simulink model "RealtimeModel"  (Simulink 7.0)
settings: Solver=FixedStepDiscrete  SolverMode=MultiTasking  StartTime=0.0  StopTime=RunningTime  FixedStep=sample  RelTol=1e-3
values from neighbouring files (symbols this model uses):
  Integrator = InitializeIntegrator(Integrator, Structure)    [RealtimeModel_Setup.m]
  SampleRate = Integrator.Timestep    [RealtimeModel_Setup.m]
  Structure = CalculateMatrices(Structure, Elements)    [RealtimeModel_Setup.m]
undefined symbols (not defined in the file or in its folder): Elements
libraries: simulink x2
(part 2 of 11)

== system RealtimeModel/Generate Element  Restoring Forces/Generate Type 3  Element Restoring Force Element 2 ==
  Displ_cmd : Inport  OutDataType=sfix(16)  OutScaling=2^0
  Constant : Constant  Value=Structure.NumFreeDOF  OutDataType=sfix(16)  OutScaling=2^0
  "Type 3 Element " : Subsystem  mask(Element Type 3){id=id}
      mask prompts: id "Element ID:"
      mask help: Enter the ID for this element corresponding with the input configuration file
  Type 3 Element RF : Stateflow chart  TreatAsAtomicUnit=on  SystemSampleTime=SampleRate
  Nodes : Outport  OutDataType=sfix(16)  OutScaling=2^0
  RF : Outport  Port=2  OutDataType=sfix(16)  OutScaling=2^0
  wires:
  Constant/1 -> Type 3 Element RF/6(NumFreeDOF)
  Displ_cmd/1 -> Type 3 Element RF/7(Displacement)
  "Type 3 Element "/1(Element) -> Type 3 Element RF/1(Element)
  Type 3 Element RF/2(RF) -> RF/1
  Type 3 Element RF/1(Nodes) -> Nodes/1
  "Type 3 Element "/2(a1) -> Type 3 Element RF/2(a1)
  "Type 3 Element "/3(a2) -> Type 3 Element RF/3(a2)
  "Type 3 Element "/4(pmx) -> Type 3 Element RF/4(pmx)
  "Type 3 Element "/5(bmy) -> Type 3 Element RF/5(bmy_init)

== system RealtimeModel/Generate Element  Restoring Forces/Generate Type 3  Element Restoring Force Element 21 ==
  Displ_cmd : Inport  OutDataType=sfix(16)  OutScaling=2^0
  Constant : Constant  Value=Structure.NumFreeDOF  OutDataType=sfix(16)  OutScaling=2^0
  "Type 3 Element " : Subsystem  mask(Element Type 3){id=id}
      mask prompts: id "Element ID:"
      mask help: Enter the ID for this element corresponding with the input configuration file
  Type 3 Element RF : Stateflow chart  TreatAsAtomicUnit=on  SystemSampleTime=SampleRate
  Nodes : Outport  OutDataType=sfix(16)  OutScaling=2^0
  RF : Outport  Port=2  OutDataType=sfix(16)  OutScaling=2^0
  wires:
  "Type 3 Element "/5(bmy) -> Type 3 Element RF/5(bmy_init)
  "Type 3 Element "/4(pmx) -> Type 3 Element RF/4(pmx)
  "Type 3 Element "/3(a2) -> Type 3 Element RF/3(a2)
  "Type 3 Element "/2(a1) -> Type 3 Element RF/2(a1)
  Type 3 Element RF/1(Nodes) -> Nodes/1
  Type 3 Element RF/2(RF) -> RF/1
  "Type 3 Element "/1(Element) -> Type 3 Element RF/1(Element)
  Displ_cmd/1 -> Type 3 Element RF/7(Displacement)
  Constant/1 -> Type 3 Element RF/6(NumFreeDOF)

== system RealtimeModel/Generate Element  Restoring Forces/Generate Type 3  Element Restoring Force Element 22 ==
  Displ_cmd : Inport  OutDataType=sfix(16)  OutScaling=2^0
  Constant : Constant  Value=Structure.NumFreeDOF  OutDataType=sfix(16)  OutScaling=2^0
  "Type 3 Element " : Subsystem  mask(Element Type 3){id=id}
      mask prompts: id "Element ID:"
      mask help: Enter the ID for this element corresponding with the input configuration file
  Type 3 Element RF : Stateflow chart  TreatAsAtomicUnit=on  SystemSampleTime=SampleRate
  Nodes : Outport  OutDataType=sfix(16)  OutScaling=2^0
  RF : Outport  Port=2  OutDataType=sfix(16)  OutScaling=2^0
  wires:
  Constant/1 -> Type 3 Element RF/6(NumFreeDOF)
  Displ_cmd/1 -> Type 3 Element RF/7(Displacement)
  "Type 3 Element "/1(Element) -> Type 3 Element RF/1(Element)
  Type 3 Element RF/2(RF) -> RF/1
  Type 3 Element RF/1(Nodes) -> Nodes/1
  "Type 3 Element "/2(a1) -> Type 3 Element RF/2(a1)
  "Type 3 Element "/3(a2) -> Type 3 Element RF/3(a2)
  "Type 3 Element "/4(pmx) -> Type 3 Element RF/4(pmx)
  "Type 3 Element "/5(bmy) -> Type 3 Element RF/5(bmy_init)

== system RealtimeModel/Generate Element  Restoring Forces/Generate Type 3  Element Restoring Force Element 24 ==
  Displ_cmd : Inport  OutDataType=sfix(16)  OutScaling=2^0
  Constant : Constant  Value=Structure.NumFreeDOF  OutDataType=sfix(16)  OutScaling=2^0
  "Type 3 Element " : Subsystem  mask(Element Type 3){id=id}
      mask prompts: id "Element ID:"
      mask help: Enter the ID for this element corresponding with the input configuration file
  Type 3 Element RF : Stateflow chart  TreatAsAtomicUnit=on  SystemSampleTime=SampleRate
  Nodes : Outport  OutDataType=sfix(16)  OutScaling=2^0
  RF : Outport  Port=2  OutDataType=sfix(16)  OutScaling=2^0
  wires:
  "Type 3 Element "/5(bmy) -> Type 3 Element RF/5(bmy_init)
  "Type 3 Element "/4(pmx) -> Type 3 Element RF/4(pmx)
  "Type 3 Element "/3(a2) -> Type 3 Element RF/3(a2)
  "Type 3 Element "/2(a1) -> Type 3 Element RF/2(a1)
  Type 3 Element RF/1(Nodes) -> Nodes/1
  Type 3 Element RF/2(RF) -> RF/1
  "Type 3 Element "/1(Element) -> Type 3 Element RF/1(Element)
  Displ_cmd/1 -> Type 3 Element RF/7(Displacement)
  Constant/1 -> Type 3 Element RF/6(NumFreeDOF)

== system RealtimeModel/Generate Element  Restoring Forces/Generate Type 3  Element Restoring Force Element 25 ==
  Displ_cmd : Inport  OutDataType=sfix(16)  OutScaling=2^0
  Constant : Constant  Value=Structure.NumFreeDOF  OutDataType=sfix(16)  OutScaling=2^0
  "Type 3 Element " : Subsystem  mask(Element Type 3){id=id}
      mask prompts: id "Element ID:"
      mask help: Enter the ID for this element corresponding with the input configuration file
  Type 3 Element RF : Stateflow chart  TreatAsAtomicUnit=on  SystemSampleTime=SampleRate
  Nodes : Outport  OutDataType=sfix(16)  OutScaling=2^0
  RF : Outport  Port=2  OutDataType=sfix(16)  OutScaling=2^0
  wires:
  "Type 3 Element "/5(bmy) -> Type 3 Element RF/5(bmy_init)
  "Type 3 Element "/4(pmx) -> Type 3 Element RF/4(pmx)
  "Type 3 Element "/3(a2) -> Type 3 Element RF/3(a2)
  "Type 3 Element "/2(a1) -> Type 3 Element RF/2(a1)
  Type 3 Element RF/1(Nodes) -> Nodes/1
  Type 3 Element RF/2(RF) -> RF/1
  "Type 3 Element "/1(Element) -> Type 3 Element RF/1(Element)
  Displ_cmd/1 -> Type 3 Element RF/7(Displacement)
  Constant/1 -> Type 3 Element RF/6(NumFreeDOF)

== system RealtimeModel/Generate Element  Restoring Forces/Generate Type 3  Element Restoring Force Element 26 ==
  Displ_cmd : Inport  OutDataType=sfix(16)  OutScaling=2^0
  Constant : Constant  Value=Structure.NumFreeDOF  OutDataType=sfix(16)  OutScaling=2^0
  "Type 3 Element " : Subsystem  mask(Element Type 3){id=id}
      mask prompts: id "Element ID:"
      mask help: Enter the ID for this element corresponding with the input configuration file
  Type 3 Element RF : Stateflow chart  TreatAsAtomicUnit=on  SystemSampleTime=SampleRate
  Nodes : Outport  OutDataType=sfix(16)  OutScaling=2^0
  RF : Outport  Port=2  OutDataType=sfix(16)  OutScaling=2^0
  wires:
  "Type 3 Element "/5(bmy) -> Type 3 Element RF/5(bmy_init)
  "Type 3 Element "/4(pmx) -> Type 3 Element RF/4(pmx)
  "Type 3 Element "/3(a2) -> Type 3 Element RF/3(a2)
  "Type 3 Element "/2(a1) -> Type 3 Element RF/2(a1)
  Type 3 Element RF/1(Nodes) -> Nodes/1
  Type 3 Element RF/2(RF) -> RF/1
  "Type 3 Element "/1(Element) -> Type 3 Element RF/1(Element)
  Displ_cmd/1 -> Type 3 Element RF/7(Displacement)
  Constant/1 -> Type 3 Element RF/6(NumFreeDOF)

== system RealtimeModel/Generate Element  Restoring Forces/Generate Type 3  Element Restoring Force Element 27 ==
  Displ_cmd : Inport  OutDataType=sfix(16)  OutScaling=2^0
  Constant : Constant  Value=Structure.NumFreeDOF  OutDataType=sfix(16)  OutScaling=2^0
  "Type 3 Element " : Subsystem  mask(Element Type 3){id=id}
      mask prompts: id "Element ID:"
      mask help: Enter the ID for this element corresponding with the input configuration file
  Type 3 Element RF : Stateflow chart  TreatAsAtomicUnit=on  SystemSampleTime=SampleRate
  Nodes : Outport  OutDataType=sfix(16)  OutScaling=2^0
  RF : Outport  Port=2  OutDataType=sfix(16)  OutScaling=2^0
  wires:
  "Type 3 Element "/5(bmy) -> Type 3 Element RF/5(bmy_init)
  "Type 3 Element "/4(pmx) -> Type 3 Element RF/4(pmx)
  "Type 3 Element "/3(a2) -> Type 3 Element RF/3(a2)
  "Type 3 Element "/2(a1) -> Type 3 Element RF/2(a1)
  Type 3 Element RF/1(Nodes) -> Nodes/1
  Type 3 Element RF/2(RF) -> RF/1
  "Type 3 Element "/1(Element) -> Type 3 Element RF/1(Element)
  Displ_cmd/1 -> Type 3 Element RF/7(Displacement)
  Constant/1 -> Type 3 Element RF/6(NumFreeDOF)

== system RealtimeModel/Generate Element  Restoring Forces/Generate Type 3  Element Restoring Force Element 30 ==
  Displ_cmd : Inport  OutDataType=sfix(16)  OutScaling=2^0
  Constant : Constant  Value=Structure.NumFreeDOF  OutDataType=sfix(16)  OutScaling=2^0
  "Type 3 Element " : Subsystem  mask(Element Type 3){id=id}
      mask prompts: id "Element ID:"
      mask help: Enter the ID for this element corresponding with the input configuration file
  Type 3 Element RF : Stateflow chart  TreatAsAtomicUnit=on  SystemSampleTime=SampleRate
  Nodes : Outport  OutDataType=sfix(16)  OutScaling=2^0
  RF : Outport  Port=2  OutDataType=sfix(16)  OutScaling=2^0
  wires:
  Constant/1 -> Type 3 Element RF/6(NumFreeDOF)
  Displ_cmd/1 -> Type 3 Element RF/7(Displacement)
  "Type 3 Element "/1(Element) -> Type 3 Element RF/1(Element)
  Type 3 Element RF/2(RF) -> RF/1
  Type 3 Element RF/1(Nodes) -> Nodes/1
  "Type 3 Element "/2(a1) -> Type 3 Element RF/2(a1)
  "Type 3 Element "/3(a2) -> Type 3 Element RF/3(a2)
  "Type 3 Element "/4(pmx) -> Type 3 Element RF/4(pmx)
  "Type 3 Element "/5(bmy) -> Type 3 Element RF/5(bmy_init)

== system RealtimeModel/Generate Element  Restoring Forces/Generate Type 3  Element Restoring Force Element 33 ==
  Displ_cmd : Inport  OutDataType=sfix(16)  OutScaling=2^0
  Constant : Constant  Value=Structure.NumFreeDOF  OutDataType=sfix(16)  OutScaling=2^0
  "Type 3 Element " : Subsystem  mask(Element Type 3){id=id}
      mask prompts: id "Element ID:"
      mask help: Enter the ID for this element corresponding with the input configuration file
  Type 3 Element RF : Stateflow chart  TreatAsAtomicUnit=on  SystemSampleTime=SampleRate
  Nodes : Outport  OutDataType=sfix(16)  OutScaling=2^0
  RF : Outport  Port=2  OutDataType=sfix(16)  OutScaling=2^0
  wires:
  Constant/1 -> Type 3 Element RF/6(NumFreeDOF)
  Displ_cmd/1 -> Type 3 Element RF/7(Displacement)
  "Type 3 Element "/1(Element) -> Type 3 Element RF/1(Element)
  Type 3 Element RF/2(RF) -> RF/1
  Type 3 Element RF/1(Nodes) -> Nodes/1
  "Type 3 Element "/2(a1) -> Type 3 Element RF/2(a1)
  "Type 3 Element "/3(a2) -> Type 3 Element RF/3(a2)
  "Type 3 Element "/4(pmx) -> Type 3 Element RF/4(pmx)
  "Type 3 Element "/5(bmy) -> Type 3 Element RF/5(bmy_init)

== system RealtimeModel/Generate Element  Restoring Forces/Generate Type 3  Element Restoring Force Element 34 ==
  Displ_cmd : Inport  OutDataType=sfix(16)  OutScaling=2^0
  Constant : Constant  Value=Structure.NumFreeDOF  OutDataType=sfix(16)  OutScaling=2^0
  "Type 3 Element " : Subsystem  mask(Element Type 3){id=id}
      mask prompts: id "Element ID:"
      mask help: Enter the ID for this element corresponding with the input configuration file
  Type 3 Element RF : Stateflow chart  TreatAsAtomicUnit=on  SystemSampleTime=SampleRate
  Nodes : Outport  OutDataType=sfix(16)  OutScaling=2^0
  RF : Outport  Port=2  OutDataType=sfix(16)  OutScaling=2^0
  wires:
  "Type 3 Element "/5(bmy) -> Type 3 Element RF/5(bmy_init)
  "Type 3 Element "/4(pmx) -> Type 3 Element RF/4(pmx)
  "Type 3 Element "/3(a2) -> Type 3 Element RF/3(a2)
  "Type 3 Element "/2(a1) -> Type 3 Element RF/2(a1)
  Type 3 Element RF/1(Nodes) -> Nodes/1
  Type 3 Element RF/2(RF) -> RF/1
  "Type 3 Element "/1(Element) -> Type 3 Element RF/1(Element)
  Displ_cmd/1 -> Type 3 Element RF/7(Displacement)
  Constant/1 -> Type 3 Element RF/6(NumFreeDOF)

== system RealtimeModel/Generate Element  Restoring Forces/Generate Type 3  Element Restoring Force Element 4 ==
  Displ_cmd : Inport  OutDataType=sfix(16)  OutScaling=2^0
  Constant : Constant  Value=Structure.NumFreeDOF  OutDataType=sfix(16)  OutScaling=2^0
  "Type 3 Element " : Subsystem  mask(Element Type 3){id=id}
      mask prompts: id "Element ID:"
      mask help: Enter the ID for this element corresponding with the input configuration file
  Type 3 Element RF : Stateflow chart  TreatAsAtomicUnit=on  SystemSampleTime=SampleRate
  Nodes : Outport  OutDataType=sfix(16)  OutScaling=2^0
  RF : Outport  Port=2  OutDataType=sfix(16)  OutScaling=2^0
  wires:
  "Type 3 Element "/5(bmy) -> Type 3 Element RF/5(bmy_init)
  "Type 3 Element "/4(pmx) -> Type 3 Element RF/4(pmx)
  "Type 3 Element "/3(a2) -> Type 3 Element RF/3(a2)
  "Type 3 Element "/2(a1) -> Type 3 Element RF/2(a1)
  Type 3 Element RF/1(Nodes) -> Nodes/1
  Type 3 Element RF/2(RF) -> RF/1
  "Type 3 Element "/1(Element) -> Type 3 Element RF/1(Element)
  Displ_cmd/1 -> Type 3 Element RF/7(Displacement)
  Constant/1 -> Type 3 Element RF/6(NumFreeDOF)

== system RealtimeModel/Generate Element  Restoring Forces/Generate Type 3  Element Restoring Force Element 5 ==
  Displ_cmd : Inport  OutDataType=sfix(16)  OutScaling=2^0
  Constant : Constant  Value=Structure.NumFreeDOF  OutDataType=sfix(16)  OutScaling=2^0
  "Type 3 Element " : Subsystem  mask(Element Type 3){id=id}
      mask prompts: id "Element ID:"
      mask help: Enter the ID for this element corresponding with the input configuration file
  Type 3 Element RF : Stateflow chart  TreatAsAtomicUnit=on  SystemSampleTime=SampleRate
  Nodes : Outport  OutDataType=sfix(16)  OutScaling=2^0
  RF : Outport  Port=2  OutDataType=sfix(16)  OutScaling=2^0
  wires:
  Constant/1 -> Type 3 Element RF/6(NumFreeDOF)
  Displ_cmd/1 -> Type 3 Element RF/7(Displacement)
  "Type 3 Element "/1(Element) -> Type 3 Element RF/1(Element)
  Type 3 Element RF/2(RF) -> RF/1
  Type 3 Element RF/1(Nodes) -> Nodes/1
  "Type 3 Element "/2(a1) -> Type 3 Element RF/2(a1)
  "Type 3 Element "/3(a2) -> Type 3 Element RF/3(a2)
  "Type 3 Element "/4(pmx) -> Type 3 Element RF/4(pmx)
  "Type 3 Element "/5(bmy) -> Type 3 Element RF/5(bmy_init)

== system RealtimeModel/Generate Element  Restoring Forces/Generate Type 3  Element Restoring Force Element 7 ==
  Displ_cmd : Inport  OutDataType=sfix(16)  OutScaling=2^0
  Constant : Constant  Value=Structure.NumFreeDOF  OutDataType=sfix(16)  OutScaling=2^0
  "Type 3 Element " : Subsystem  mask(Element Type 3){id=id}
      mask prompts: id "Element ID:"
      mask help: Enter the ID for this element corresponding with the input configuration file
  Type 3 Element RF : Stateflow chart  TreatAsAtomicUnit=on  SystemSampleTime=SampleRate
  Nodes : Outport  OutDataType=sfix(16)  OutScaling=2^0
  RF : Outport  Port=2  OutDataType=sfix(16)  OutScaling=2^0
  wires:
  "Type 3 Element "/5(bmy) -> Type 3 Element RF/5(bmy_init)
  "Type 3 Element "/4(pmx) -> Type 3 Element RF/4(pmx)
  "Type 3 Element "/3(a2) -> Type 3 Element RF/3(a2)
  "Type 3 Element "/2(a1) -> Type 3 Element RF/2(a1)
  Type 3 Element RF/1(Nodes) -> Nodes/1
  Type 3 Element RF/2(RF) -> RF/1
  "Type 3 Element "/1(Element) -> Type 3 Element RF/1(Element)
  Displ_cmd/1 -> Type 3 Element RF/7(Displacement)
  Constant/1 -> Type 3 Element RF/6(NumFreeDOF)

== system RealtimeModel/Generate Element  Restoring Forces/Generate Type 3  Element Restoring Force Element 8 ==
  Displ_cmd : Inport  OutDataType=sfix(16)  OutScaling=2^0
  Constant : Constant  Value=Structure.NumFreeDOF  OutDataType=sfix(16)  OutScaling=2^0
  "Type 3 Element " : Subsystem  mask(Element Type 3){id=id}
      mask prompts: id "Element ID:"
      mask help: Enter the ID for this element corresponding with the input configuration file
  Type 3 Element RF : Stateflow chart  TreatAsAtomicUnit=on  SystemSampleTime=SampleRate
  Nodes : Outport  OutDataType=sfix(16)  OutScaling=2^0
  RF : Outport  Port=2  OutDataType=sfix(16)  OutScaling=2^0
  wires:
  Constant/1 -> Type 3 Element RF/6(NumFreeDOF)
  Displ_cmd/1 -> Type 3 Element RF/7(Displacement)
  "Type 3 Element "/1(Element) -> Type 3 Element RF/1(Element)
  Type 3 Element RF/2(RF) -> RF/1
  Type 3 Element RF/1(Nodes) -> Nodes/1
  "Type 3 Element "/2(a1) -> Type 3 Element RF/2(a1)
  "Type 3 Element "/3(a2) -> Type 3 Element RF/3(a2)
  "Type 3 Element "/4(pmx) -> Type 3 Element RF/4(pmx)
  "Type 3 Element "/5(bmy) -> Type 3 Element RF/5(bmy_init)

== system RealtimeModel/Generate Element  Restoring Forces/Generate Type 3  Element Restoring Force Element 9 ==
  Displ_cmd : Inport  OutDataType=sfix(16)  OutScaling=2^0
  Constant : Constant  Value=Structure.NumFreeDOF  OutDataType=sfix(16)  OutScaling=2^0
  "Type 3 Element " : Subsystem  mask(Element Type 3){id=id}
      mask prompts: id "Element ID:"
      mask help: Enter the ID for this element corresponding with the input configuration file
  Type 3 Element RF : Stateflow chart  TreatAsAtomicUnit=on  SystemSampleTime=SampleRate
  Nodes : Outport  OutDataType=sfix(16)  OutScaling=2^0
  RF : Outport  Port=2  OutDataType=sfix(16)  OutScaling=2^0
  wires:
  "Type 3 Element "/5(bmy) -> Type 3 Element RF/5(bmy_init)
  "Type 3 Element "/4(pmx) -> Type 3 Element RF/4(pmx)
  "Type 3 Element "/3(a2) -> Type 3 Element RF/3(a2)
  "Type 3 Element "/2(a1) -> Type 3 Element RF/2(a1)
  Type 3 Element RF/1(Nodes) -> Nodes/1
  Type 3 Element RF/2(RF) -> RF/1
  "Type 3 Element "/1(Element) -> Type 3 Element RF/1(Element)
  Displ_cmd/1 -> Type 3 Element RF/7(Displacement)
  Constant/1 -> Type 3 Element RF/6(NumFreeDOF)

== system RealtimeModel/Generate Element  Restoring Forces/Generate Type 4  Element Restoring Force Element 35  ==
  Displ_cmd : Inport  OutDataType=sfix(16)  OutScaling=2^0
  Constant : Constant  Value=Structure.NumFreeDOF  OutDataType=sfix(16)  OutScaling=2^0
  "Type 4 Element " : Subsystem  mask(Element Type 4){id=id}
      mask prompts: id "Element ID:"
      mask help: Enter the ID for this element corresponding with the input configuration file
  Type 4 Element RF : Stateflow chart  TreatAsAtomicUnit=on  SystemSampleTime=SampleRate
  Nodes : Outport  OutDataType=sfix(16)  OutScaling=2^0
  RF : Outport  Port=2  OutDataType=sfix(16)  OutScaling=2^0
  wires:
  "Type 4 Element "/1(Element) -> Type 4 Element RF/1(Element)
  Type 4 Element RF/1(Nodes) -> Nodes/1
  Type 4 Element RF/2(RF) -> RF/1
  Constant/1 -> Type 4 Element RF/2(NumFreeDOF)
  Displ_cmd/1 -> Type 4 Element RF/3(Displacement)

== system RealtimeModel/Generate Element  Restoring Forces/Generate Type 1  Element Restoring Force Element 11/Type 1 Element  ==
  Bus Creator : BusCreator  Inputs=13
  Data Store Memory10 : DataStoreMemory  DataStoreName=MaterialE  InitialValue=Elements{id}.Material(1).E  OutDataType=sfix(16)  OutScaling=2^0
  Data Store Memory11 : DataStoreMemory  DataStoreName=Inertia  InitialValue=Elements{id}.Inertia  OutDataType=sfix(16)  OutScaling=2^0
  Data Store Memory12 : DataStoreMemory  DataStoreName=Area  InitialValue=Elements{id}.Area  OutDataType=sfix(16)  OutScaling=2^0
  Data Store Memory13 : DataStoreMemory  DataStoreName=Node2UX  InitialValue=Elements{id}.Nodes(2).UX  OutDataType=sfix(16)  OutScaling=2^0
  Data Store Memory14 : DataStoreMemory  DataStoreName=Node1THETA  InitialValue=Elements{id}.Nodes(1).THETA  OutDataType=sfix(16)  OutScaling=2^0
  Data Store Memory15 : DataStoreMemory  DataStoreName=Node2UY  InitialValue=Elements{id}.Nodes(2).UY  OutDataType=sfix(16)  OutScaling=2^0
  Data Store Memory2 : DataStoreMemory  DataStoreName=Node1Xcoord  InitialValue=Elements{id}.Nodes(1).Xcoord  OutDataType=sfix(16)  OutScaling=2^0
  Data Store Memory3 : DataStoreMemory  DataStoreName=Node1Ycoord  InitialValue=Elements{id}.Nodes(1).Ycoord  OutDataType=sfix(16)  OutScaling=2^0
  Data Store Memory4 : DataStoreMemory  DataStoreName=Node1UX  InitialValue=Elements{id}.Nodes(1).UX  OutDataType=sfix(16)  OutScaling=2^0
  Data Store Memory6 : DataStoreMemory  DataStoreName=Node2Xcoord  InitialValue=Elements{id}.Nodes(2).Xcoord  OutDataType=sfix(16)  OutScaling=2^0
  Data Store Memory7 : DataStoreMemory  DataStoreName=Node2Ycoord  InitialValue=Elements{id}.Nodes(2).Ycoord  OutDataType=sfix(16)  OutScaling=2^0
  Data Store Memory8 : DataStoreMemory  DataStoreName=Node2THETA  InitialValue=Elements{id}.Nodes(2).THETA  OutDataType=sfix(16)  OutScaling=2^0
  Data Store Memory9 : DataStoreMemory  DataStoreName=Node1UY  InitialValue=Elements{id}.Nodes(1).UY  OutDataType=sfix(16)  OutScaling=2^0
  Data Store Read1 : DataStoreRead  DataStoreName=Node1UX  SampleTime=-1
  Data Store Read10 : DataStoreRead  DataStoreName=MaterialE  SampleTime=-1
  Data Store Read11 : DataStoreRead  DataStoreName=Area  SampleTime=-1
  Data Store Read12 : DataStoreRead  DataStoreName=Inertia  SampleTime=-1
  Data Store Read13 : DataStoreRead  DataStoreName=Node2UY  SampleTime=-1
  Data Store Read14 : DataStoreRead  DataStoreName=Node2THETA  SampleTime=-1
  Data Store Read2 : DataStoreRead  DataStoreName=Node1Xcoord  SampleTime=-1
  Data Store Read3 : DataStoreRead  DataStoreName=Node1Ycoord  SampleTime=-1
  Data Store Read4 : DataStoreRead  DataStoreName=Node1UY  SampleTime=-1
  Data Store Read6 : DataStoreRead  DataStoreName=Node2Xcoord  SampleTime=-1
  Data Store Read7 : DataStoreRead  DataStoreName=Node2Ycoord  SampleTime=-1
  Data Store Read8 : DataStoreRead  DataStoreName=Node1THETA  SampleTime=-1
  Data Store Read9 : DataStoreRead  DataStoreName=Node2UX  SampleTime=-1
  Element : Outport  OutDataType=sfix(16)  OutScaling=2^0
  wires:
  Bus Creator/1 -> Element/1
  Data Store Read12/1 -> Bus Creator/7  "Inertia"
  Data Store Read11/1 -> Bus Creator/6  "Area"
  Data Store Read10/1 -> Bus Creator/5  "Material E"
  Data Store Read7/1 -> Bus Creator/4  "Node2 Ycoord"
  Data Store Read6/1 -> Bus Creator/3  "Node2 Xcoord"
  Data Store Read3/1 -> Bus Creator/2  "Node1 Ycoord"
  Data Store Read2/1 -> Bus Creator/1  "Node1 Xcoord"
  Data Store Read1/1 -> Bus Creator/8  "Node1UX"
  Data Store Read4/1 -> Bus Creator/9
  Data Store Read8/1 -> Bus Creator/10
  Data Store Read9/1 -> Bus Creator/11
  Data Store Read13/1 -> Bus Creator/12
  Data Store Read14/1 -> Bus Creator/13

== system RealtimeModel/Generate Element  Restoring Forces/Generate Type 1  Element Restoring Force Element 12/Type 1 Element  ==
  Bus Creator : BusCreator  Inputs=13
  Data Store Memory10 : DataStoreMemory  DataStoreName=MaterialE  InitialValue=Elements{id}.Material(1).E  OutDataType=sfix(16)  OutScaling=2^0
  Data Store Memory11 : DataStoreMemory  DataStoreName=Inertia  InitialValue=Elements{id}.Inertia  OutDataType=sfix(16)  OutScaling=2^0
  Data Store Memory12 : DataStoreMemory  DataStoreName=Area  InitialValue=Elements{id}.Area  OutDataType=sfix(16)  OutScaling=2^0
  Data Store Memory13 : DataStoreMemory  DataStoreName=Node2UX  InitialValue=Elements{id}.Nodes(2).UX  OutDataType=sfix(16)  OutScaling=2^0
  Data Store Memory14 : DataStoreMemory  DataStoreName=Node1THETA  InitialValue=Elements{id}.Nodes(1).THETA  OutDataType=sfix(16)  OutScaling=2^0
  Data Store Memory15 : DataStoreMemory  DataStoreName=Node2UY  InitialValue=Elements{id}.Nodes(2).UY  OutDataType=sfix(16)  OutScaling=2^0
  Data Store Memory2 : DataStoreMemory  DataStoreName=Node1Xcoord  InitialValue=Elements{id}.Nodes(1).Xcoord  OutDataType=sfix(16)  OutScaling=2^0
  Data Store Memory3 : DataStoreMemory  DataStoreName=Node1Ycoord  InitialValue=Elements{id}.Nodes(1).Ycoord  OutDataType=sfix(16)  OutScaling=2^0
  Data Store Memory4 : DataStoreMemory  DataStoreName=Node1UX  InitialValue=Elements{id}.Nodes(1).UX  OutDataType=sfix(16)  OutScaling=2^0
  Data Store Memory6 : DataStoreMemory  DataStoreName=Node2Xcoord  InitialValue=Elements{id}.Nodes(2).Xcoord  OutDataType=sfix(16)  OutScaling=2^0
  Data Store Memory7 : DataStoreMemory  DataStoreName=Node2Ycoord  InitialValue=Elements{id}.Nodes(2).Ycoord  OutDataType=sfix(16)  OutScaling=2^0
  Data Store Memory8 : DataStoreMemory  DataStoreName=Node2THETA  InitialValue=Elements{id}.Nodes(2).THETA  OutDataType=sfix(16)  OutScaling=2^0
  Data Store Memory9 : DataStoreMemory  DataStoreName=Node1UY  InitialValue=Elements{id}.Nodes(1).UY  OutDataType=sfix(16)  OutScaling=2^0
  Data Store Read1 : DataStoreRead  DataStoreName=Node1UX  SampleTime=-1
  Data Store Read10 : DataStoreRead  DataStoreName=MaterialE  SampleTime=-1
  Data Store Read11 : DataStoreRead  DataStoreName=Area  SampleTime=-1
  Data Store Read12 : DataStoreRead  DataStoreName=Inertia  SampleTime=-1
  Data Store Read13 : DataStoreRead  DataStoreName=Node2UY  SampleTime=-1
  Data Store Read14 : DataStoreRead  DataStoreName=Node2THETA  SampleTime=-1
  Data Store Read2 : DataStoreRead  DataStoreName=Node1Xcoord  SampleTime=-1
  Data Store Read3 : DataStoreRead  DataStoreName=Node1Ycoord  SampleTime=-1
  Data Store Read4 : DataStoreRead  DataStoreName=Node1UY  SampleTime=-1
  Data Store Read6 : DataStoreRead  DataStoreName=Node2Xcoord  SampleTime=-1
  Data Store Read7 : DataStoreRead  DataStoreName=Node2Ycoord  SampleTime=-1
  Data Store Read8 : DataStoreRead  DataStoreName=Node1THETA  SampleTime=-1
  Data Store Read9 : DataStoreRead  DataStoreName=Node2UX  SampleTime=-1
  Element : Outport  OutDataType=sfix(16)  OutScaling=2^0
  wires:
  Data Store Read14/1 -> Bus Creator/13
  Data Store Read13/1 -> Bus Creator/12
  Data Store Read9/1 -> Bus Creator/11
  Data Store Read8/1 -> Bus Creator/10
  Data Store Read4/1 -> Bus Creator/9
  Data Store Read1/1 -> Bus Creator/8  "Node1UX"
  Data Store Read2/1 -> Bus Creator/1  "Node1 Xcoord"
  Data Store Read3/1 -> Bus Creator/2  "Node1 Ycoord"
  Data Store Read6/1 -> Bus Creator/3  "Node2 Xcoord"
  Data Store Read7/1 -> Bus Creator/4  "Node2 Ycoord"
  Data Store Read10/1 -> Bus Creator/5  "Material E"
  Data Store Read11/1 -> Bus Creator/6  "Area"
  Data Store Read12/1 -> Bus Creator/7  "Inertia"
  Bus Creator/1 -> Element/1

== system RealtimeModel/Generate Element  Restoring Forces/Generate Type 1  Element Restoring Force Element 14/Type 1 Element  ==
  Bus Creator : BusCreator  Inputs=13
  Data Store Memory10 : DataStoreMemory  DataStoreName=MaterialE  InitialValue=Elements{id}.Material(1).E  OutDataType=sfix(16)  OutScaling=2^0
  Data Store Memory11 : DataStoreMemory  DataStoreName=Inertia  InitialValue=Elements{id}.Inertia  OutDataType=sfix(16)  OutScaling=2^0
  Data Store Memory12 : DataStoreMemory  DataStoreName=Area  InitialValue=Elements{id}.Area  OutDataType=sfix(16)  OutScaling=2^0
  Data Store Memory13 : DataStoreMemory  DataStoreName=Node2UX  InitialValue=Elements{id}.Nodes(2).UX  OutDataType=sfix(16)  OutScaling=2^0
  Data Store Memory14 : DataStoreMemory  DataStoreName=Node1THETA  InitialValue=Elements{id}.Nodes(1).THETA  OutDataType=sfix(16)  OutScaling=2^0
  Data Store Memory15 : DataStoreMemory  DataStoreName=Node2UY  InitialValue=Elements{id}.Nodes(2).UY  OutDataType=sfix(16)  OutScaling=2^0
  Data Store Memory2 : DataStoreMemory  DataStoreName=Node1Xcoord  InitialValue=Elements{id}.Nodes(1).Xcoord  OutDataType=sfix(16)  OutScaling=2^0
  Data Store Memory3 : DataStoreMemory  DataStoreName=Node1Ycoord  InitialValue=Elements{id}.Nodes(1).Ycoord  OutDataType=sfix(16)  OutScaling=2^0
  Data Store Memory4 : DataStoreMemory  DataStoreName=Node1UX  InitialValue=Elements{id}.Nodes(1).UX  OutDataType=sfix(16)  OutScaling=2^0
  Data Store Memory6 : DataStoreMemory  DataStoreName=Node2Xcoord  InitialValue=Elements{id}.Nodes(2).Xcoord  OutDataType=sfix(16)  OutScaling=2^0
  Data Store Memory7 : DataStoreMemory  DataStoreName=Node2Ycoord  InitialValue=Elements{id}.Nodes(2).Ycoord  OutDataType=sfix(16)  OutScaling=2^0
  Data Store Memory8 : DataStoreMemory  DataStoreName=Node2THETA  InitialValue=Elements{id}.Nodes(2).THETA  OutDataType=sfix(16)  OutScaling=2^0
  Data Store Memory9 : DataStoreMemory  DataStoreName=Node1UY  InitialValue=Elements{id}.Nodes(1).UY  OutDataType=sfix(16)  OutScaling=2^0
  Data Store Read1 : DataStoreRead  DataStoreName=Node1UX  SampleTime=-1
  Data Store Read10 : DataStoreRead  DataStoreName=MaterialE  SampleTime=-1
  Data Store Read11 : DataStoreRead  DataStoreName=Area  SampleTime=-1
  Data Store Read12 : DataStoreRead  DataStoreName=Inertia  SampleTime=-1
  Data Store Read13 : DataStoreRead  DataStoreName=Node2UY  SampleTime=-1
  Data Store Read14 : DataStoreRead  DataStoreName=Node2THETA  SampleTime=-1
  Data Store Read2 : DataStoreRead  DataStoreName=Node1Xcoord  SampleTime=-1
  Data Store Read3 : DataStoreRead  DataStoreName=Node1Ycoord  SampleTime=-1
  Data Store Read4 : DataStoreRead  DataStoreName=Node1UY  SampleTime=-1
  Data Store Read6 : DataStoreRead  DataStoreName=Node2Xcoord  SampleTime=-1
  Data Store Read7 : DataStoreRead  DataStoreName=Node2Ycoord  SampleTime=-1
  Data Store Read8 : DataStoreRead  DataStoreName=Node1THETA  SampleTime=-1
  Data Store Read9 : DataStoreRead  DataStoreName=Node2UX  SampleTime=-1
  Element : Outport  OutDataType=sfix(16)  OutScaling=2^0
  wires:
  Bus Creator/1 -> Element/1
  Data Store Read12/1 -> Bus Creator/7  "Inertia"
  Data Store Read11/1 -> Bus Creator/6  "Area"
  Data Store Read10/1 -> Bus Creator/5  "Material E"
  Data Store Read7/1 -> Bus Creator/4  "Node2 Ycoord"
  Data Store Read6/1 -> Bus Creator/3  "Node2 Xcoord"
  Data Store Read3/1 -> Bus Creator/2  "Node1 Ycoord"
  Data Store Read2/1 -> Bus Creator/1  "Node1 Xcoord"
  Data Store Read1/1 -> Bus Creator/8  "Node1UX"
  Data Store Read4/1 -> Bus Creator/9
  Data Store Read8/1 -> Bus Creator/10
  Data Store Read9/1 -> Bus Creator/11
  Data Store Read13/1 -> Bus Creator/12
  Data Store Read14/1 -> Bus Creator/13

== system RealtimeModel/Generate Element  Restoring Forces/Generate Type 1  Element Restoring Force Element 15/Type 1 Element  ==
  Bus Creator : BusCreator  Inputs=13
  Data Store Memory10 : DataStoreMemory  DataStoreName=MaterialE  InitialValue=Elements{id}.Material(1).E  OutDataType=sfix(16)  OutScaling=2^0
  Data Store Memory11 : DataStoreMemory  DataStoreName=Inertia  InitialValue=Elements{id}.Inertia  OutDataType=sfix(16)  OutScaling=2^0
  Data Store Memory12 : DataStoreMemory  DataStoreName=Area  InitialValue=Elements{id}.Area  OutDataType=sfix(16)  OutScaling=2^0
  Data Store Memory13 : DataStoreMemory  DataStoreName=Node2UX  InitialValue=Elements{id}.Nodes(2).UX  OutDataType=sfix(16)  OutScaling=2^0
  Data Store Memory14 : DataStoreMemory  DataStoreName=Node1THETA  InitialValue=Elements{id}.Nodes(1).THETA  OutDataType=sfix(16)  OutScaling=2^0
  Data Store Memory15 : DataStoreMemory  DataStoreName=Node2UY  InitialValue=Elements{id}.Nodes(2).UY  OutDataType=sfix(16)  OutScaling=2^0
  Data Store Memory2 : DataStoreMemory  DataStoreName=Node1Xcoord  InitialValue=Elements{id}.Nodes(1).Xcoord  OutDataType=sfix(16)  OutScaling=2^0
  Data Store Memory3 : DataStoreMemory  DataStoreName=Node1Ycoord  InitialValue=Elements{id}.Nodes(1).Ycoord  OutDataType=sfix(16)  OutScaling=2^0
  Data Store Memory4 : DataStoreMemory  DataStoreName=Node1UX  InitialValue=Elements{id}.Nodes(1).UX  OutDataType=sfix(16)  OutScaling=2^0
  Data Store Memory6 : DataStoreMemory  DataStoreName=Node2Xcoord  InitialValue=Elements{id}.Nodes(2).Xcoord  OutDataType=sfix(16)  OutScaling=2^0
  Data Store Memory7 : DataStoreMemory  DataStoreName=Node2Ycoord  InitialValue=Elements{id}.Nodes(2).Ycoord  OutDataType=sfix(16)  OutScaling=2^0
  Data Store Memory8 : DataStoreMemory  DataStoreName=Node2THETA  InitialValue=Elements{id}.Nodes(2).THETA  OutDataType=sfix(16)  OutScaling=2^0
  Data Store Memory9 : DataStoreMemory  DataStoreName=Node1UY  InitialValue=Elements{id}.Nodes(1).UY  OutDataType=sfix(16)  OutScaling=2^0
  Data Store Read1 : DataStoreRead  DataStoreName=Node1UX  SampleTime=-1
  Data Store Read10 : DataStoreRead  DataStoreName=MaterialE  SampleTime=-1
  Data Store Read11 : DataStoreRead  DataStoreName=Area  SampleTime=-1
  Data Store Read12 : DataStoreRead  DataStoreName=Inertia  SampleTime=-1
  Data Store Read13 : DataStoreRead  DataStoreName=Node2UY  SampleTime=-1
  Data Store Read14 : DataStoreRead  DataStoreName=Node2THETA  SampleTime=-1
  Data Store Read2 : DataStoreRead  DataStoreName=Node1Xcoord  SampleTime=-1
  Data Store Read3 : DataStoreRead  DataStoreName=Node1Ycoord  SampleTime=-1
  Data Store Read4 : DataStoreRead  DataStoreName=Node1UY  SampleTime=-1
  Data Store Read6 : DataStoreRead  DataStoreName=Node2Xcoord  SampleTime=-1
  Data Store Read7 : DataStoreRead  DataStoreName=Node2Ycoord  SampleTime=-1
  Data Store Read8 : DataStoreRead  DataStoreName=Node1THETA  SampleTime=-1
  Data Store Read9 : DataStoreRead  DataStoreName=Node2UX  SampleTime=-1
  Element : Outport  OutDataType=sfix(16)  OutScaling=2^0
  wires:
  Data Store Read14/1 -> Bus Creator/13
  Data Store Read13/1 -> Bus Creator/12
  Data Store Read9/1 -> Bus Creator/11
  Data Store Read8/1 -> Bus Creator/10
  Data Store Read4/1 -> Bus Creator/9
  Data Store Read1/1 -> Bus Creator/8  "Node1UX"
  Data Store Read2/1 -> Bus Creator/1  "Node1 Xcoord"
  Data Store Read3/1 -> Bus Creator/2  "Node1 Ycoord"
  Data Store Read6/1 -> Bus Creator/3  "Node2 Xcoord"
  Data Store Read7/1 -> Bus Creator/4  "Node2 Ycoord"
  Data Store Read10/1 -> Bus Creator/5  "Material E"
  Data Store Read11/1 -> Bus Creator/6  "Area"
  Data Store Read12/1 -> Bus Creator/7  "Inertia"
  Bus Creator/1 -> Element/1

== system RealtimeModel/Generate Element  Restoring Forces/Generate Type 1  Element Restoring Force Element 28/Type 1 Element  ==
  Bus Creator : BusCreator  Inputs=13
  Data Store Memory10 : DataStoreMemory  DataStoreName=MaterialE  InitialValue=Elements{id}.Material(1).E  OutDataType=sfix(16)  OutScaling=2^0
  Data Store Memory11 : DataStoreMemory  DataStoreName=Inertia  InitialValue=Elements{id}.Inertia  OutDataType=sfix(16)  OutScaling=2^0
  Data Store Memory12 : DataStoreMemory  DataStoreName=Area  InitialValue=Elements{id}.Area  OutDataType=sfix(16)  OutScaling=2^0
  Data Store Memory13 : DataStoreMemory  DataStoreName=Node2UX  InitialValue=Elements{id}.Nodes(2).UX  OutDataType=sfix(16)  OutScaling=2^0
  Data Store Memory14 : DataStoreMemory  DataStoreName=Node1THETA  InitialValue=Elements{id}.Nodes(1).THETA  OutDataType=sfix(16)  OutScaling=2^0
  Data Store Memory15 : DataStoreMemory  DataStoreName=Node2UY  InitialValue=Elements{id}.Nodes(2).UY  OutDataType=sfix(16)  OutScaling=2^0
  Data Store Memory2 : DataStoreMemory  DataStoreName=Node1Xcoord  InitialValue=Elements{id}.Nodes(1).Xcoord  OutDataType=sfix(16)  OutScaling=2^0
  Data Store Memory3 : DataStoreMemory  DataStoreName=Node1Ycoord  InitialValue=Elements{id}.Nodes(1).Ycoord  OutDataType=sfix(16)  OutScaling=2^0
  Data Store Memory4 : DataStoreMemory  DataStoreName=Node1UX  InitialValue=Elements{id}.Nodes(1).UX  OutDataType=sfix(16)  OutScaling=2^0
  Data Store Memory6 : DataStoreMemory  DataStoreName=Node2Xcoord  InitialValue=Elements{id}.Nodes(2).Xcoord  OutDataType=sfix(16)  OutScaling=2^0
  Data Store Memory7 : DataStoreMemory  DataStoreName=Node2Ycoord  InitialValue=Elements{id}.Nodes(2).Ycoord  OutDataType=sfix(16)  OutScaling=2^0
  Data Store Memory8 : DataStoreMemory  DataStoreName=Node2THETA  InitialValue=Elements{id}.Nodes(2).THETA  OutDataType=sfix(16)  OutScaling=2^0
  Data Store Memory9 : DataStoreMemory  DataStoreName=Node1UY  InitialValue=Elements{id}.Nodes(1).UY  OutDataType=sfix(16)  OutScaling=2^0
  Data Store Read1 : DataStoreRead  DataStoreName=Node1UX  SampleTime=-1
  Data Store Read10 : DataStoreRead  DataStoreName=MaterialE  SampleTime=-1
  Data Store Read11 : DataStoreRead  DataStoreName=Area  SampleTime=-1
  Data Store Read12 : DataStoreRead  DataStoreName=Inertia  SampleTime=-1
  Data Store Read13 : DataStoreRead  DataStoreName=Node2UY  SampleTime=-1
  Data Store Read14 : DataStoreRead  DataStoreName=Node2THETA  SampleTime=-1
  Data Store Read2 : DataStoreRead  DataStoreName=Node1Xcoord  SampleTime=-1
  Data Store Read3 : DataStoreRead  DataStoreName=Node1Ycoord  SampleTime=-1
  Data Store Read4 : DataStoreRead  DataStoreName=Node1UY  SampleTime=-1
  Data Store Read6 : DataStoreRead  DataStoreName=Node2Xcoord  SampleTime=-1
  Data Store Read7 : DataStoreRead  DataStoreName=Node2Ycoord  SampleTime=-1
  Data Store Read8 : DataStoreRead  DataStoreName=Node1THETA  SampleTime=-1
  Data Store Read9 : DataStoreRead  DataStoreName=Node2UX  SampleTime=-1
  Element : Outport  OutDataType=sfix(16)  OutScaling=2^0
  wires:
  Bus Creator/1 -> Element/1
  Data Store Read12/1 -> Bus Creator/7  "Inertia"
  Data Store Read11/1 -> Bus Creator/6  "Area"
  Data Store Read10/1 -> Bus Creator/5  "Material E"
  Data Store Read7/1 -> Bus Creator/4  "Node2 Ycoord"
  Data Store Read6/1 -> Bus Creator/3  "Node2 Xcoord"
  Data Store Read3/1 -> Bus Creator/2  "Node1 Ycoord"
  Data Store Read2/1 -> Bus Creator/1  "Node1 Xcoord"
  Data Store Read1/1 -> Bus Creator/8  "Node1UX"
  Data Store Read4/1 -> Bus Creator/9
  Data Store Read8/1 -> Bus Creator/10
  Data Store Read9/1 -> Bus Creator/11
  Data Store Read13/1 -> Bus Creator/12
  Data Store Read14/1 -> Bus Creator/13

== system RealtimeModel/Generate Element  Restoring Forces/Generate Type 1  Element Restoring Force Element 29/Type 1 Element  ==
  Bus Creator : BusCreator  Inputs=13
  Data Store Memory10 : DataStoreMemory  DataStoreName=MaterialE  InitialValue=Elements{id}.Material(1).E  OutDataType=sfix(16)  OutScaling=2^0
  Data Store Memory11 : DataStoreMemory  DataStoreName=Inertia  InitialValue=Elements{id}.Inertia  OutDataType=sfix(16)  OutScaling=2^0
  Data Store Memory12 : DataStoreMemory  DataStoreName=Area  InitialValue=Elements{id}.Area  OutDataType=sfix(16)  OutScaling=2^0
  Data Store Memory13 : DataStoreMemory  DataStoreName=Node2UX  InitialValue=Elements{id}.Nodes(2).UX  OutDataType=sfix(16)  OutScaling=2^0
  Data Store Memory14 : DataStoreMemory  DataStoreName=Node1THETA  InitialValue=Elements{id}.Nodes(1).THETA  OutDataType=sfix(16)  OutScaling=2^0
  Data Store Memory15 : DataStoreMemory  DataStoreName=Node2UY  InitialValue=Elements{id}.Nodes(2).UY  OutDataType=sfix(16)  OutScaling=2^0
  Data Store Memory2 : DataStoreMemory  DataStoreName=Node1Xcoord  InitialValue=Elements{id}.Nodes(1).Xcoord  OutDataType=sfix(16)  OutScaling=2^0
  Data Store Memory3 : DataStoreMemory  DataStoreName=Node1Ycoord  InitialValue=Elements{id}.Nodes(1).Ycoord  OutDataType=sfix(16)  OutScaling=2^0
  Data Store Memory4 : DataStoreMemory  DataStoreName=Node1UX  InitialValue=Elements{id}.Nodes(1).UX  OutDataType=sfix(16)  OutScaling=2^0
  Data Store Memory6 : DataStoreMemory  DataStoreName=Node2Xcoord  InitialValue=Elements{id}.Nodes(2).Xcoord  OutDataType=sfix(16)  OutScaling=2^0
  Data Store Memory7 : DataStoreMemory  DataStoreName=Node2Ycoord  InitialValue=Elements{id}.Nodes(2).Ycoord  OutDataType=sfix(16)  OutScaling=2^0
  Data Store Memory8 : DataStoreMemory  DataStoreName=Node2THETA  InitialValue=Elements{id}.Nodes(2).THETA  OutDataType=sfix(16)  OutScaling=2^0
  Data Store Memory9 : DataStoreMemory  DataStoreName=Node1UY  InitialValue=Elements{id}.Nodes(1).UY  OutDataType=sfix(16)  OutScaling=2^0
  Data Store Read1 : DataStoreRead  DataStoreName=Node1UX  SampleTime=-1
  Data Store Read10 : DataStoreRead  DataStoreName=MaterialE  SampleTime=-1
  Data Store Read11 : DataStoreRead  DataStoreName=Area  SampleTime=-1
  Data Store Read12 : DataStoreRead  DataStoreName=Inertia  SampleTime=-1
  Data Store Read13 : DataStoreRead  DataStoreName=Node2UY  SampleTime=-1
  Data Store Read14 : DataStoreRead  DataStoreName=Node2THETA  SampleTime=-1
  Data Store Read2 : DataStoreRead  DataStoreName=Node1Xcoord  SampleTime=-1
  Data Store Read3 : DataStoreRead  DataStoreName=Node1Ycoord  SampleTime=-1
  Data Store Read4 : DataStoreRead  DataStoreName=Node1UY  SampleTime=-1
  Data Store Read6 : DataStoreRead  DataStoreName=Node2Xcoord  SampleTime=-1
  Data Store Read7 : DataStoreRead  DataStoreName=Node2Ycoord  SampleTime=-1
  Data Store Read8 : DataStoreRead  DataStoreName=Node1THETA  SampleTime=-1
  Data Store Read9 : DataStoreRead  DataStoreName=Node2UX  SampleTime=-1
  Element : Outport  OutDataType=sfix(16)  OutScaling=2^0
  wires:
  Data Store Read14/1 -> Bus Creator/13
  Data Store Read13/1 -> Bus Creator/12
  Data Store Read9/1 -> Bus Creator/11
  Data Store Read8/1 -> Bus Creator/10
  Data Store Read4/1 -> Bus Creator/9
  Data Store Read1/1 -> Bus Creator/8  "Node1UX"
  Data Store Read2/1 -> Bus Creator/1  "Node1 Xcoord"
  Data Store Read3/1 -> Bus Creator/2  "Node1 Ycoord"
  Data Store Read6/1 -> Bus Creator/3  "Node2 Xcoord"
  Data Store Read7/1 -> Bus Creator/4  "Node2 Ycoord"
  Data Store Read10/1 -> Bus Creator/5  "Material E"
  Data Store Read11/1 -> Bus Creator/6  "Area"
  Data Store Read12/1 -> Bus Creator/7  "Inertia"
  Bus Creator/1 -> Element/1

== system RealtimeModel/Generate Element  Restoring Forces/Generate Type 1  Element Restoring Force Element 31/Type 1 Element  ==
  Bus Creator : BusCreator  Inputs=13
  Data Store Memory10 : DataStoreMemory  DataStoreName=MaterialE  InitialValue=Elements{id}.Material(1).E  OutDataType=sfix(16)  OutScaling=2^0
  Data Store Memory11 : DataStoreMemory  DataStoreName=Inertia  InitialValue=Elements{id}.Inertia  OutDataType=sfix(16)  OutScaling=2^0
  Data Store Memory12 : DataStoreMemory  DataStoreName=Area  InitialValue=Elements{id}.Area  OutDataType=sfix(16)  OutScaling=2^0
  Data Store Memory13 : DataStoreMemory  DataStoreName=Node2UX  InitialValue=Elements{id}.Nodes(2).UX  OutDataType=sfix(16)  OutScaling=2^0
  Data Store Memory14 : DataStoreMemory  DataStoreName=Node1THETA  InitialValue=Elements{id}.Nodes(1).THETA  OutDataType=sfix(16)  OutScaling=2^0
  Data Store Memory15 : DataStoreMemory  DataStoreName=Node2UY  InitialValue=Elements{id}.Nodes(2).UY  OutDataType=sfix(16)  OutScaling=2^0
  Data Store Memory2 : DataStoreMemory  DataStoreName=Node1Xcoord  InitialValue=Elements{id}.Nodes(1).Xcoord  OutDataType=sfix(16)  OutScaling=2^0
  Data Store Memory3 : DataStoreMemory  DataStoreName=Node1Ycoord  InitialValue=Elements{id}.Nodes(1).Ycoord  OutDataType=sfix(16)  OutScaling=2^0
  Data Store Memory4 : DataStoreMemory  DataStoreName=Node1UX  InitialValue=Elements{id}.Nodes(1).UX  OutDataType=sfix(16)  OutScaling=2^0
  Data Store Memory6 : DataStoreMemory  DataStoreName=Node2Xcoord  InitialValue=Elements{id}.Nodes(2).Xcoord  OutDataType=sfix(16)  OutScaling=2^0
  Data Store Memory7 : DataStoreMemory  DataStoreName=Node2Ycoord  InitialValue=Elements{id}.Nodes(2).Ycoord  OutDataType=sfix(16)  OutScaling=2^0
  Data Store Memory8 : DataStoreMemory  DataStoreName=Node2THETA  InitialValue=Elements{id}.Nodes(2).THETA  OutDataType=sfix(16)  OutScaling=2^0
  Data Store Memory9 : DataStoreMemory  DataStoreName=Node1UY  InitialValue=Elements{id}.Nodes(1).UY  OutDataType=sfix(16)  OutScaling=2^0
  Data Store Read1 : DataStoreRead  DataStoreName=Node1UX  SampleTime=-1
  Data Store Read10 : DataStoreRead  DataStoreName=MaterialE  SampleTime=-1
  Data Store Read11 : DataStoreRead  DataStoreName=Area  SampleTime=-1
  Data Store Read12 : DataStoreRead  DataStoreName=Inertia  SampleTime=-1
  Data Store Read13 : DataStoreRead  DataStoreName=Node2UY  SampleTime=-1
  Data Store Read14 : DataStoreRead  DataStoreName=Node2THETA  SampleTime=-1
  Data Store Read2 : DataStoreRead  DataStoreName=Node1Xcoord  SampleTime=-1
  Data Store Read3 : DataStoreRead  DataStoreName=Node1Ycoord  SampleTime=-1
  Data Store Read4 : DataStoreRead  DataStoreName=Node1UY  SampleTime=-1
  Data Store Read6 : DataStoreRead  DataStoreName=Node2Xcoord  SampleTime=-1
  Data Store Read7 : DataStoreRead  DataStoreName=Node2Ycoord  SampleTime=-1
  Data Store Read8 : DataStoreRead  DataStoreName=Node1THETA  SampleTime=-1
  Data Store Read9 : DataStoreRead  DataStoreName=Node2UX  SampleTime=-1
  Element : Outport  OutDataType=sfix(16)  OutScaling=2^0
  wires:
  Bus Creator/1 -> Element/1
  Data Store Read12/1 -> Bus Creator/7  "Inertia"
  Data Store Read11/1 -> Bus Creator/6  "Area"
  Data Store Read10/1 -> Bus Creator/5  "Material E"
  Data Store Read7/1 -> Bus Creator/4  "Node2 Ycoord"
  Data Store Read6/1 -> Bus Creator/3  "Node2 Xcoord"
  Data Store Read3/1 -> Bus Creator/2  "Node1 Ycoord"
  Data Store Read2/1 -> Bus Creator/1  "Node1 Xcoord"
  Data Store Read1/1 -> Bus Creator/8  "Node1UX"
  Data Store Read4/1 -> Bus Creator/9
  Data Store Read8/1 -> Bus Creator/10
  Data Store Read9/1 -> Bus Creator/11
  Data Store Read13/1 -> Bus Creator/12
  Data Store Read14/1 -> Bus Creator/13

== system RealtimeModel/Generate Element  Restoring Forces/Generate Type 1  Element Restoring Force Element 32/Type 1 Element  ==
  Bus Creator : BusCreator  Inputs=13
  Data Store Memory10 : DataStoreMemory  DataStoreName=MaterialE  InitialValue=Elements{id}.Material(1).E  OutDataType=sfix(16)  OutScaling=2^0
  Data Store Memory11 : DataStoreMemory  DataStoreName=Inertia  InitialValue=Elements{id}.Inertia  OutDataType=sfix(16)  OutScaling=2^0
  Data Store Memory12 : DataStoreMemory  DataStoreName=Area  InitialValue=Elements{id}.Area  OutDataType=sfix(16)  OutScaling=2^0
  Data Store Memory13 : DataStoreMemory  DataStoreName=Node2UX  InitialValue=Elements{id}.Nodes(2).UX  OutDataType=sfix(16)  OutScaling=2^0
  Data Store Memory14 : DataStoreMemory  DataStoreName=Node1THETA  InitialValue=Elements{id}.Nodes(1).THETA  OutDataType=sfix(16)  OutScaling=2^0
  Data Store Memory15 : DataStoreMemory  DataStoreName=Node2UY  InitialValue=Elements{id}.Nodes(2).UY  OutDataType=sfix(16)  OutScaling=2^0
  Data Store Memory2 : DataStoreMemory  DataStoreName=Node1Xcoord  InitialValue=Elements{id}.Nodes(1).Xcoord  OutDataType=sfix(16)  OutScaling=2^0
  Data Store Memory3 : DataStoreMemory  DataStoreName=Node1Ycoord  InitialValue=Elements{id}.Nodes(1).Ycoord  OutDataType=sfix(16)  OutScaling=2^0
  Data Store Memory4 : DataStoreMemory  DataStoreName=Node1UX  InitialValue=Elements{id}.Nodes(1).UX  OutDataType=sfix(16)  OutScaling=2^0
  Data Store Memory6 : DataStoreMemory  DataStoreName=Node2Xcoord  InitialValue=Elements{id}.Nodes(2).Xcoord  OutDataType=sfix(16)  OutScaling=2^0
  Data Store Memory7 : DataStoreMemory  DataStoreName=Node2Ycoord  InitialValue=Elements{id}.Nodes(2).Ycoord  OutDataType=sfix(16)  OutScaling=2^0
  Data Store Memory8 : DataStoreMemory  DataStoreName=Node2THETA  InitialValue=Elements{id}.Nodes(2).THETA  OutDataType=sfix(16)  OutScaling=2^0
  Data Store Memory9 : DataStoreMemory  DataStoreName=Node1UY  InitialValue=Elements{id}.Nodes(1).UY  OutDataType=sfix(16)  OutScaling=2^0
  Data Store Read1 : DataStoreRead  DataStoreName=Node1UX  SampleTime=-1
  Data Store Read10 : DataStoreRead  DataStoreName=MaterialE  SampleTime=-1
  Data Store Read11 : DataStoreRead  DataStoreName=Area  SampleTime=-1
  Data Store Read12 : DataStoreRead  DataStoreName=Inertia  SampleTime=-1
  Data Store Read13 : DataStoreRead  DataStoreName=Node2UY  SampleTime=-1
  Data Store Read14 : DataStoreRead  DataStoreName=Node2THETA  SampleTime=-1
  Data Store Read2 : DataStoreRead  DataStoreName=Node1Xcoord  SampleTime=-1
  Data Store Read3 : DataStoreRead  DataStoreName=Node1Ycoord  SampleTime=-1
  Data Store Read4 : DataStoreRead  DataStoreName=Node1UY  SampleTime=-1
  Data Store Read6 : DataStoreRead  DataStoreName=Node2Xcoord  SampleTime=-1
  Data Store Read7 : DataStoreRead  DataStoreName=Node2Ycoord  SampleTime=-1
  Data Store Read8 : DataStoreRead  DataStoreName=Node1THETA  SampleTime=-1
  Data Store Read9 : DataStoreRead  DataStoreName=Node2UX  SampleTime=-1
  Element : Outport  OutDataType=sfix(16)  OutScaling=2^0
  wires:
  Data Store Read14/1 -> Bus Creator/13
  Data Store Read13/1 -> Bus Creator/12
  Data Store Read9/1 -> Bus Creator/11
  Data Store Read8/1 -> Bus Creator/10
  Data Store Read4/1 -> Bus Creator/9
  Data Store Read1/1 -> Bus Creator/8  "Node1UX"
  Data Store Read2/1 -> Bus Creator/1  "Node1 Xcoord"
  Data Store Read3/1 -> Bus Creator/2  "Node1 Ycoord"
  Data Store Read6/1 -> Bus Creator/3  "Node2 Xcoord"
  Data Store Read7/1 -> Bus Creator/4  "Node2 Ycoord"
  Data Store Read10/1 -> Bus Creator/5  "Material E"
  Data Store Read11/1 -> Bus Creator/6  "Area"
  Data Store Read12/1 -> Bus Creator/7  "Inertia"
  Bus Creator/1 -> Element/1
